simulink model "project_first_try_simulink"  (R2021a)
settings: Solver=VariableStepAuto  StartTime=0.0  StopTime=0.5  RelTol=1e-3
libraries: commdigbbndpm3 x6, commanapbnd3 x6, visionsources x1
settings Model: Creator=manami  LastModifiedBy=manami

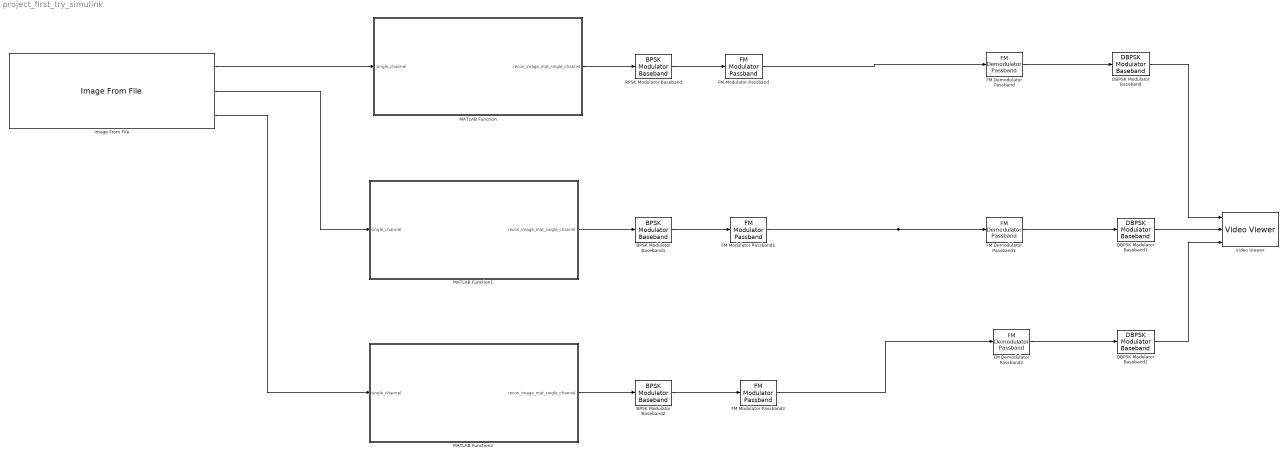
== system project_first_try_simulink ==
  BPSK Modulator Baseband : commdigbbndpm3/BPSK Modulator Baseband  Ph=0  outDtype=double  outWordLen=16  outUDDataType=sfix(16)  outFracLenMode=Best precision  outFracLen=15  outDataTypeStr=double  outLastDataTypeStr=double
  BPSK Modulator Baseband1 : commdigbbndpm3/BPSK Modulator Baseband  Ph=0  outDtype=double  outWordLen=16  outUDDataType=sfix(16)  outFracLenMode=Best precision  outFracLen=15  outDataTypeStr=double  outLastDataTypeStr=double
  BPSK Modulator Baseband2 : commdigbbndpm3/BPSK Modulator Baseband  Ph=0  outDtype=double  outWordLen=16  outUDDataType=sfix(16)  outFracLenMode=Best precision  outFracLen=15  outDataTypeStr=double  outLastDataTypeStr=double
  DBPSK Modulator Baseband : commdigbbndpm3/DBPSK Modulator Baseband  Ph=0  outDtype=double
      settings: SourceProductBaseCode=CM
  DBPSK Modulator Baseband1 : commdigbbndpm3/DBPSK Modulator Baseband  Ph=0  outDtype=double
      settings: SourceProductBaseCode=CM
  DBPSK Modulator Baseband2 : commdigbbndpm3/DBPSK Modulator Baseband  Ph=0  outDtype=double
      settings: SourceProductBaseCode=CM
  FM Demodulator Passband : commanapbnd3/FM Demodulator Passband  Fc=300  Ph=0  Kc=50  Ho=100
      settings: SourceProductBaseCode=CM
  FM Demodulator Passband1 : commanapbnd3/FM Demodulator Passband  Fc=3000  Ph=0  Kc=500  Ho=100
      settings: SourceProductBaseCode=CM
  FM Demodulator Passband2 : commanapbnd3/FM Demodulator Passband  Fc=30000  Ph=0  Kc=5000  Ho=100
      settings: SourceProductBaseCode=CM
  FM Modulator Passband : commanapbnd3/FM Modulator Passband  Fc=300  Ph=0  Kc=50
      settings: SourceProductBaseCode=CM
  FM Modulator Passband1 : commanapbnd3/FM Modulator Passband  Fc=3000  Ph=0  Kc=500
      settings: SourceProductBaseCode=CM
  FM Modulator Passband2 : commanapbnd3/FM Modulator Passband  Fc=30000  Ph=0  Kc=5000
      settings: SourceProductBaseCode=CM
  Image From File : visionsources/Image From File  Tag=vipblks_nd  FileName=D:\com project\174423899_808724736692372_8447064076947490794_n.jpg  Ts=inf  imagePorts=Separate color signals  OutPortLabels=R|G|B  ImageDataType=Inherit from input image  sdImageDataType=uint(8)  Signed=on  WordLength=16  FractionLengthMode=User-defined  FractionLength=15
  MATLAB Function : MATLAB Function  TreatAsAtomicUnit=on
  MATLAB Function1 : MATLAB Function  TreatAsAtomicUnit=on
  MATLAB Function2 : MATLAB Function  TreatAsAtomicUnit=on
  Video Viewer : VideoViewer  imagePorts=separate color signals  FigPos=[2041 741 418 304]
  wires:
  Image From File/1 -> MATLAB Function/1(single_channel)
  MATLAB Function/1(recon_image_mat_single_channel) -> BPSK Modulator Baseband/1
  Image From File/2 -> MATLAB Function1/1(single_channel)
  MATLAB Function1/1(recon_image_mat_single_channel) -> BPSK Modulator Baseband1/1
  Image From File/3 -> MATLAB Function2/1(single_channel)
  MATLAB Function2/1(recon_image_mat_single_channel) -> BPSK Modulator Baseband2/1
  BPSK Modulator Baseband/1 -> FM Modulator Passband/1
  BPSK Modulator Baseband1/1 -> FM Modulator Passband1/1
  BPSK Modulator Baseband2/1 -> FM Modulator Passband2/1
  FM Modulator Passband/1 -> FM Demodulator Passband/1
  FM Modulator Passband1/1 -> FM Demodulator Passband1/1
  FM Modulator Passband2/1 -> FM Demodulator Passband2/1
  FM Demodulator Passband/1 -> DBPSK Modulator Baseband/1
  FM Demodulator Passband1/1 -> DBPSK Modulator Baseband1/1
  FM Demodulator Passband2/1 -> DBPSK Modulator Baseband2/1
  DBPSK Modulator Baseband/1 -> Video Viewer/1
  DBPSK Modulator Baseband1/1 -> Video Viewer/2
  DBPSK Modulator Baseband2/1 -> Video Viewer/3

== matlab function project_first_try_simulink/MATLAB Function ==
  data: single_channel input; recon_image_mat_single_channel output
function recon_image_mat_single_channel = single_channel_image_read(single_channel)
%#codegen
row = length(single_channel(:,1));
col = length(single_channel);
bin = zeros(1,row*col);;
k=1;
for i=1:row
    bin(1,k:k+col-1) = single_channel(i,:);
    k = k+col;
end
binla = dec2bin(bin);
bintemp = binla;
bintemp(:,7:8) = '0';
new = bin2dec(bintemp)';
recon = zeros(row,col);
for i = 1:row
    recon(i,1:col) = new(1,col*(i-1)+1:col*i);
end 
newimage = recon;
recon_image_mat_single_channel = cast(newimage,'uint8');

== matlab function project_first_try_simulink/MATLAB Function2 ==
  data: single_channel input; recon_image_mat_single_channel output
function recon_image_mat_single_channel = single_channel_image_read(single_channel)
%#codegen
row = length(single_channel(:,1));
col = length(single_channel);
bin = zeros(1,row*col);;
k=1;
for i=1:row
    bin(1,k:k+col-1) = single_channel(i,:);
    k = k+col;
end
binla = dec2bin(bin);
bintemp = binla;
bintemp(:,7:8) = '0';
new = bin2dec(bintemp)';
recon = zeros(row,col);
for i = 1:row
    recon(i,1:col) = new(1,col*(i-1)+1:col*i);
end 
newimage = recon;
recon_image_mat_single_channel = cast(newimage,'uint8');

== matlab function project_first_try_simulink/MATLAB Function1 ==
  data: single_channel input; recon_image_mat_single_channel output
function recon_image_mat_single_channel = single_channel_image_read(single_channel)
%#codegen
row = length(single_channel(:,1));
col = length(single_channel);
bin = zeros(1,row*col);;
k=1;
for i=1:row
    bin(1,k:k+col-1) = single_channel(i,:);
    k = k+col;
end
binla = dec2bin(bin);
bintemp = binla;
bintemp(:,7:8) = '0';
new = bin2dec(bintemp)';
recon = zeros(row,col);
for i = 1:row
    recon(i,1:col) = new(1,col*(i-1)+1:col*i);
end 
newimage = recon;
recon_image_mat_single_channel = cast(newimage,'uint8');
